simulink model "first_session"  (R2021a)
settings: Solver=VariableStepAuto  StartTime=0.0  StopTime=10.0  RelTol=1e-3
settings Model: Creator=Beshary  LastModifiedBy=Beshary

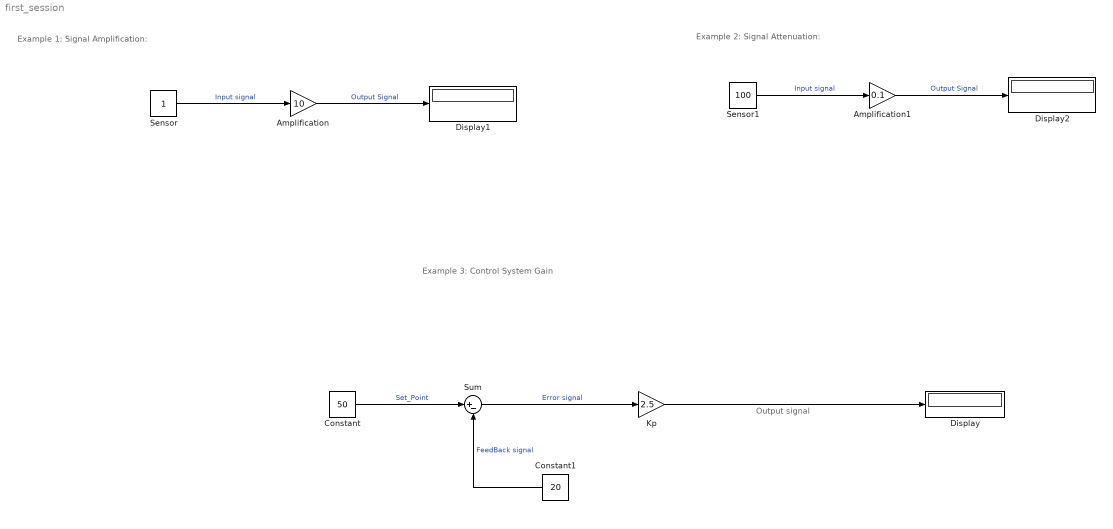
== system first_session ==
  note: Output signal
  note: Example 3: Control System Gain
  note: Example 2: Signal Attenuation:
  note: Example 1: Signal Amplification:
  Amplification : Gain  Gain=10
  Amplification1 : Gain  Gain=0.1
  Constant : Constant  Value=50
  Constant1 : Constant  Value=20
  Display : Display
  Display1 : Display
  Display2 : Display
  Kp : Gain  Gain=2.5
  Sensor : Constant
  Sensor1 : Constant  Value=100
  Sum : Sum  Inputs=|+-
  wires:
  Sum/1 -> Kp/1  "Error signal"
  Constant/1 -> Sum/1  "Set_Point"
  Kp/1 -> Display/1
  Sensor/1 -> Amplification/1  "Input signal"
  Amplification/1 -> Display1/1  "Output Signal"
  Amplification1/1 -> Display2/1  "Output Signal"
  Sensor1/1 -> Amplification1/1  "Input signal"
  Constant1/1 -> Sum/2  "FeedBack signal"
